simulink model "DC_Motor_Control"  (R2020b)
settings: Solver=FixedStepAuto  StartTime=0.0  StopTime=tTot  FixedStep=TsSim  RelTol=1e-6  EnableMultiTasking=on
InitFcn:
  | pid_init
StopFcn:
  | pid_plot
values from neighbouring files (symbols this model uses):
  a1 = Taud/(Taud+Ts)    (= 0.5)    [pid_init.m]
  AntiWindup = 0    [pid_init.m]
  b0 = Ts/(Taud+Ts)    (= 0.5)    [pid_init.m]
  Bm = 0.01    [pid_init.m]
  Jm = 0.0015    [pid_init.m]
  ka = 0.1    [pid_init.m]
  Kb = 0.03    [pid_init.m]
  kd = 0.008    [pid_init.m]
  ki = 5.7    [pid_init.m]
  Km = 0.04    [pid_init.m]
  kp = 0.7    [pid_init.m]
  L = 0.02    [pid_init.m]
  R = 1    [pid_init.m]
  Taud = 0.01    [pid_init.m]
  Ts = 0.01    [pid_init.m]
  umax = 12    [pid_init.m]
  umin = -12    [pid_init.m]
  xStep = 10    [pid_init.m]
settings Model: Creator=Pixelated  LastModifiedBy=U00EBN1
settings DataIOCC: ReturnWorkspaceOutputs=off
settings OptimizationCC: LifeSpan=inf
settings DebuggingCC: IgnoredZcDiagnostic=none  SFUnexpectedBacktrackingDiag=warning  SFNoUnconditionalDefaultTransitionDiag=warning  SFExecutionAtInitializationDiag=none  ArithmeticOperatorsInVariantConditions=warning
settings SFSimCC: SimUseLocalCustomCode=off  CustomCodeUndefinedFunction=UseInterfaceOnly
settings RTWCC: RTWUseLocalCustomCode=off
settings CodeAppCC: StateflowObjectComments=on
settings GRTTargetCC: TargetLangStandard=C89/C90 (ANSI)
settings ConfigComp: CovMetricSettings=dw  CovSaveCumulativeToWorkspaceVar=on  CovSaveSingleToWorkspaceVar=on  CovExternalEMLEnable=off

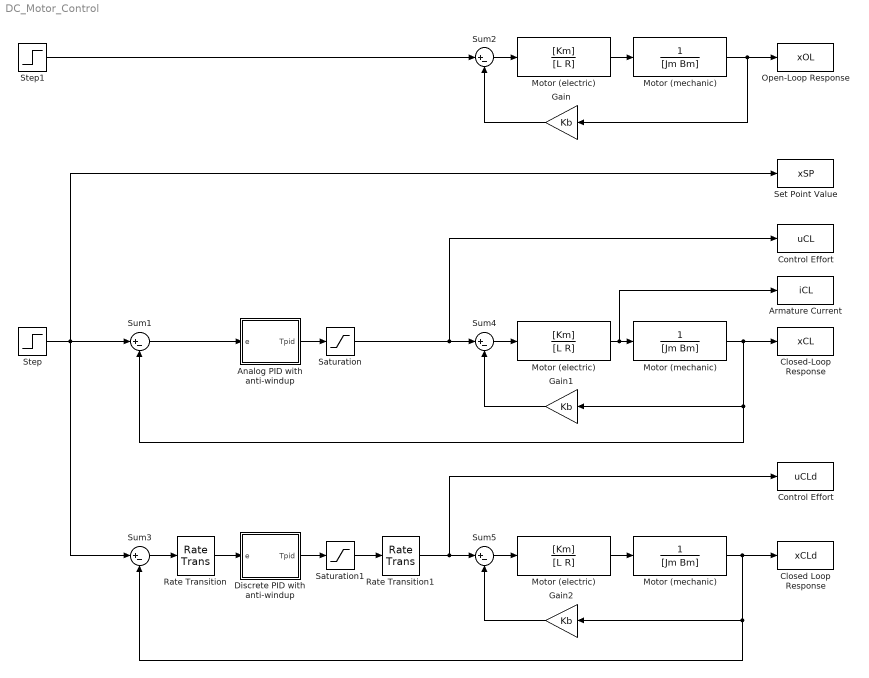
== system DC_Motor_Control ==
  Analog PID with anti-windup : Subsystem
  Armature Current : ToWorkspace  VariableName=iCL  SampleTime=-1
  "Closed Loop Response " : ToWorkspace  VariableName=xCLd  SampleTime=-1
  Closed-Loop Response : ToWorkspace  VariableName=xCL  SampleTime=-1
  Control Effort : ToWorkspace  VariableName=uCL  SampleTime=-1
  "Control Effort " : ToWorkspace  VariableName=uCLd  SampleTime=-1
  Discrete PID with anti-windup : Subsystem
  Gain : Gain  Gain=Kb
  Gain1 : Gain  Gain=Kb
  Gain2 : Gain  Gain=Kb
  Motor (electric) : TransferFcn  Numerator=[Km]  Denominator=[L R]
  "Motor (electric) " : TransferFcn  Numerator=[Km]  Denominator=[L R]
  "Motor (electric)  " : TransferFcn  Numerator=[Km]  Denominator=[L R]
  Motor (mechanic) : TransferFcn  Denominator=[Jm Bm]
  "Motor (mechanic) " : TransferFcn  Denominator=[Jm Bm]
  "Motor (mechanic)  " : TransferFcn  Denominator=[Jm Bm]
  Open-Loop Response : ToWorkspace  VariableName=xOL  SampleTime=-1
  Rate Transition : RateTransition  OutPortSampleTime=Ts
  Rate Transition1 : RateTransition
  Saturation : Saturate  UpperLimit=umax  LowerLimit=umin  ZeroCross=off
  Saturation1 : Saturate  UpperLimit=umax  LowerLimit=umin
  Set Point Value : ToWorkspace  VariableName=xSP  SampleTime=-1
  Step : Step  Time=0.1  After=xStep  SampleTime=0
  Step1 : Step  Time=0.1  After=xStep/(Km/(R*Bm+Kb*Km))  SampleTime=0
  Sum{1..5} (5 alike) : Sum  Inputs=|+-
  wires:
  "Motor (mechanic) "/1 -> Closed-Loop Response/1, Gain1/1, Sum1/2
  Saturation/1 -> Sum4/1, Control Effort/1
  Sum1/1 -> Analog PID with anti-windup/1(e)
  Analog PID with anti-windup/1(Tpid) -> Saturation/1
  Sum3/1 -> Rate Transition/1
  Saturation1/1 -> Rate Transition1/1
  Discrete PID with anti-windup/1(Tpid) -> Saturation1/1
  Rate Transition/1 -> Discrete PID with anti-windup/1(e)
  "Motor (mechanic)  "/1 -> "Closed Loop Response "/1, Gain2/1, Sum3/2
  Step/1 -> Set Point Value/1, Sum3/1, Sum1/1
  Rate Transition1/1 -> Sum5/1, "Control Effort "/1
  Motor (electric)/1 -> Motor (mechanic)/1
  Motor (mechanic)/1 -> Open-Loop Response/1, Gain/1
  Sum2/1 -> Motor (electric)/1
  Step1/1 -> Sum2/1
  Gain/1 -> Sum2/2
  Gain1/1 -> Sum4/2
  Sum4/1 -> "Motor (electric) "/1
  "Motor (electric) "/1 -> Armature Current/1, "Motor (mechanic) "/1
  Sum5/1 -> "Motor (electric)  "/1
  "Motor (electric)  "/1 -> "Motor (mechanic)  "/1
  Gain2/1 -> Sum5/2

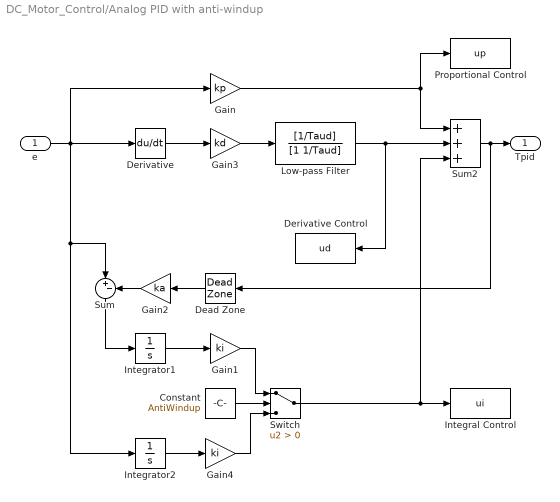
== system DC_Motor_Control/Analog PID with anti-windup ==
  e : Inport
  Constant : Constant  Value=AntiWindup
  Dead Zone : DeadZone  LowerValue=umin  UpperValue=umax  ZeroCross=off  SaturateOnIntegerOverflow=on
  Derivative : Derivative
  Derivative Control : ToWorkspace  VariableName=ud
  Gain : Gain  Gain=kp
  Gain1 : Gain  Gain=ki
  Gain2 : Gain  Gain=ka
  Gain3 : Gain  Gain=kd
  Gain4 : Gain  Gain=ki
  Integral Control : ToWorkspace  VariableName=ui
  Integrator1 : Integrator
  Integrator2 : Integrator
  Low-pass Filter : TransferFcn  Numerator=[1/Taud]  Denominator=[1 1/Taud]
  Proportional Control : ToWorkspace  VariableName=up
  Sum : Sum  Inputs=|+-
  Sum2 : Sum  Inputs=+++
  Switch : Switch  Criteria=u2 > Threshold
  Tpid : Outport
  wires:
  Switch/1 -> Integral Control/1, Sum2/3
  Integrator2/1 -> Gain4/1
  Dead Zone/1 -> Gain2/1
  Gain/1 -> Sum2/1, Proportional Control/1
  Integrator1/1 -> Gain1/1
  Derivative/1 -> Gain3/1
  e/1 -> Derivative/1, Gain/1, Integrator2/1, Sum/1
  Sum2/1 -> Tpid/1, Dead Zone/1
  Constant/1 -> Switch/2
  Gain4/1 -> Switch/3
  Gain1/1 -> Switch/1
  Sum/1 -> Integrator1/1
  Gain2/1 -> Sum/2
  Gain3/1 -> Low-pass Filter/1
  Low-pass Filter/1 -> Sum2/2, Derivative Control/1

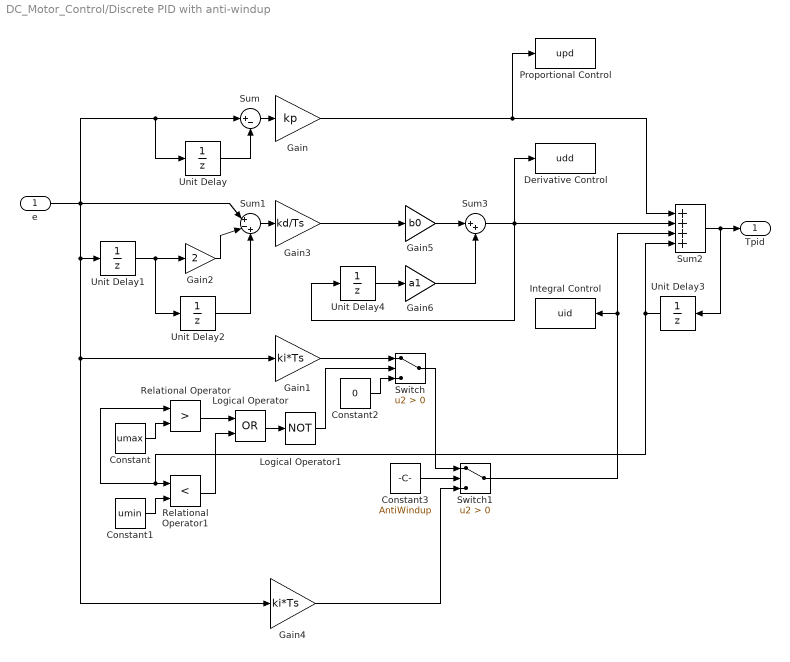
== system DC_Motor_Control/Discrete PID with anti-windup ==
  e : Inport
  Constant : Constant  Value=umax
  Constant1 : Constant  Value=umin
  Constant2 : Constant  Value=0
  Constant3 : Constant  Value=AntiWindup
  Derivative Control : ToWorkspace  VariableName=udd  SampleTime=-1
  Gain : Gain  Gain=kp
  Gain1 : Gain  Gain=ki*Ts
  Gain2 : Gain  Gain=2
  Gain3 : Gain  Gain=kd/Ts
  Gain4 : Gain  Gain=ki*Ts
  Gain5 : Gain  Gain=b0
  Gain6 : Gain  Gain=a1
  Integral Control : ToWorkspace  VariableName=uid  SampleTime=-1
  Logical Operator : Logic  Operator=OR  AllPortsSameDT=off  OutDataTypeStr=boolean
  Logical Operator1 : Logic  Operator=NOT  AllPortsSameDT=off  OutDataTypeStr=boolean
  Proportional Control : ToWorkspace  VariableName=upd  SampleTime=-1
  Relational Operator : RelationalOperator  Operator=>  OutDataTypeStr=boolean  RndMeth=Nearest
  Relational Operator1 : RelationalOperator  Operator=<  OutDataTypeStr=boolean  RndMeth=Nearest
  Sum : Sum  Inputs=|+-
  Sum1 : Sum  Inputs=|+-+
  Sum2 : Sum  Inputs=++++
  Sum3 : Sum  Inputs=|++
  Switch : Switch  Criteria=u2 > Threshold
  Switch1 : Switch  Criteria=u2 > Threshold
  Unit Delay{,1..4} (5 alike) : UnitDelay  SampleTime=-1  HasFrameUpgradeWarning=on
  Tpid : Outport
  wires:
  Switch1/1 -> Sum2/3, Integral Control/1
  Sum/1 -> Gain/1
  e/1 -> Sum1/1, Unit Delay1/1, Gain4/1, Gain1/1, Sum/1, Unit Delay/1
  Unit Delay/1 -> Sum/2
  Unit Delay1/1 -> Gain2/1, Unit Delay2/1
  Gain2/1 -> Sum1/2
  Unit Delay2/1 -> Sum1/3
  Sum1/1 -> Gain3/1
  Sum2/1 -> Tpid/1, Unit Delay3/1
  Gain1/1 -> Switch/1
  Gain/1 -> Proportional Control/1, Sum2/1
  Unit Delay3/1 -> Sum2/4, Relational Operator/1, Relational Operator1/1
  Constant2/1 -> Switch/3
  Logical Operator1/1 -> Switch/2
  Constant/1 -> Relational Operator/2
  Constant1/1 -> Relational Operator1/2
  Relational Operator/1 -> Logical Operator/1
  Relational Operator1/1 -> Logical Operator/2
  Logical Operator/1 -> Logical Operator1/1
  Switch/1 -> Switch1/1
  Constant3/1 -> Switch1/2
  Gain4/1 -> Switch1/3
  Gain3/1 -> Gain5/1
  Gain5/1 -> Sum3/1
  Sum3/1 -> Derivative Control/1, Unit Delay4/1, Sum2/2
  Unit Delay4/1 -> Gain6/1
  Gain6/1 -> Sum3/2
